simulink model "s_adrc_2"  (R2020b)
settings: Solver=VariableStepAuto  StartTime=0.0  StopTime=10
settings Model: Creator=Amir  LastModifiedBy=Amir
settings DataIOCC: ReturnWorkspaceOutputs=off

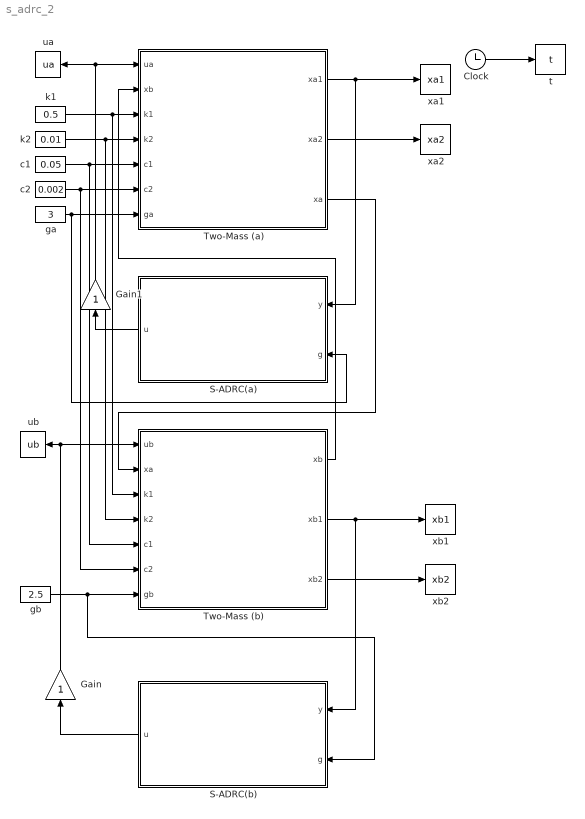
== system s_adrc_2 ==
  Clock : Clock
  Gain : Gain
  Gain1 : Gain
  S-ADRC(a) : Subsystem  mask{alpha1=3, alpha2=3, alpha3=1, epsilon=0.05, xhat0=[1;2;0], p=1, rho=0.5, beta=4, delta=1e+6, deltap=1e+6}
      mask prompts: xhat0 "xhat(0):"; deltap "delta_prime:"
      mask DialogControl ParameterGroupVar Prompt: LESO Parameters
      mask DialogControl ParameterGroupVar_copy Prompt: Controller Parameters
      mask DialogControl ParameterGroupVar_copy_copy Prompt: Thresholds
  S-ADRC(b) : Subsystem  mask{alpha1=3, alpha2=3, alpha3=1, epsilon=0.05, xhat0=[1;2;0], p=1, rho=0.5, beta=4, delta=1e+6, deltap=1e+6}
      mask prompts: xhat0 "xhat(0):"; deltap "delta_prime:"
      mask DialogControl ParameterGroupVar Prompt: LESO Parameters
      mask DialogControl ParameterGroupVar_copy Prompt: Controller Parameters
      mask DialogControl ParameterGroupVar_copy_copy Prompt: Thresholds
  Two-Mass (a) : Subsystem  mask{x0=[1.5;0.5]}
      mask prompts: x0 "x(0):"
  Two-Mass (b) : Subsystem  mask{x0=[1;2]}
      mask prompts: x0 "x(0):"
  c1 : Constant  Value=0.05
  c2 : Constant  Value=0.002
  ga : Constant  Value=3
  gb : Constant  Value=2.5
  k1 : Constant  Value=0.5
  k2 : Constant  Value=0.01
  t : ToWorkspace  VariableName=t  SampleTime=-1
      settings: Save2DSignal=2-D array (concatenate along first dimension)
  ua : ToWorkspace  VariableName=ua  SampleTime=-1
      settings: Save2DSignal=2-D array (concatenate along first dimension)
  ub : ToWorkspace  VariableName=ub  SampleTime=-1
      settings: Save2DSignal=2-D array (concatenate along first dimension)
  xa1 : ToWorkspace  VariableName=xa1  SampleTime=-1
      settings: Save2DSignal=2-D array (concatenate along first dimension)
  xa2 : ToWorkspace  VariableName=xa2  SampleTime=-1
      settings: Save2DSignal=2-D array (concatenate along first dimension)
  xb1 : ToWorkspace  VariableName=xb1  SampleTime=-1
      settings: Save2DSignal=2-D array (concatenate along first dimension)
  xb2 : ToWorkspace  VariableName=xb2  SampleTime=-1
      settings: Save2DSignal=2-D array (concatenate along first dimension)
  wires:
  Two-Mass (a)/2(xa2) -> xa2/1
  Clock/1 -> t/1
  Two-Mass (a)/1(xa1) -> S-ADRC(a)/1(y), xa1/1
  S-ADRC(a)/1(u) -> Gain1/1
  S-ADRC(b)/1(u) -> Gain/1
  Two-Mass (b)/3(xb2) -> xb2/1
  Two-Mass (b)/2(xb1) -> S-ADRC(b)/1(y), xb1/1
  Two-Mass (b)/1(xb) -> Two-Mass (a)/2(xb)
  Two-Mass (a)/3(xa) -> Two-Mass (b)/2(xa)
  k1/1 -> Two-Mass (b)/3(k1), Two-Mass (a)/3(k1)
  k2/1 -> Two-Mass (b)/4(k2), Two-Mass (a)/4(k2)
  c1/1 -> Two-Mass (b)/5(c1), Two-Mass (a)/5(c1)
  c2/1 -> Two-Mass (b)/6(c2), Two-Mass (a)/6(c2)
  ga/1 -> S-ADRC(a)/2(g), Two-Mass (a)/7(ga)
  gb/1 -> S-ADRC(b)/2(g), Two-Mass (b)/7(gb)
  Gain/1 -> Two-Mass (b)/1(ub), ub/1
  Gain1/1 -> Two-Mass (a)/1(ua), ua/1

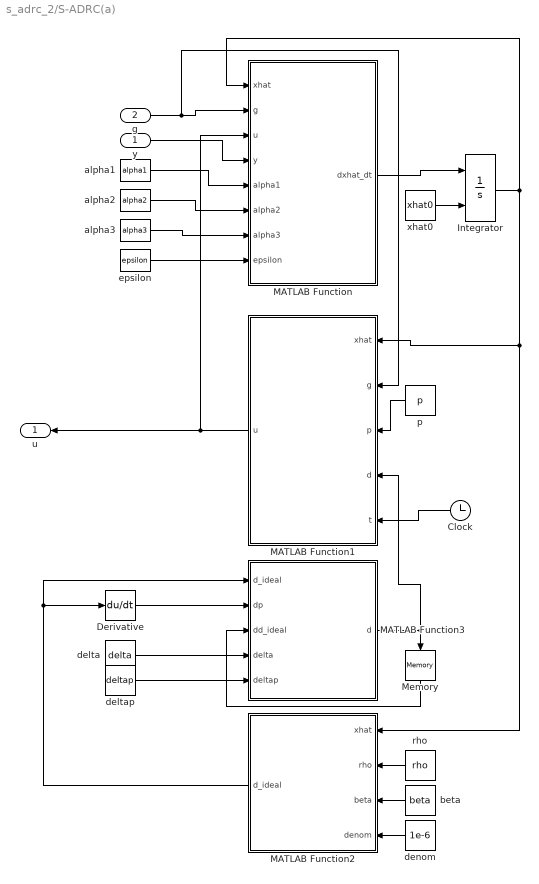
== system s_adrc_2/S-ADRC(a) ==
  y : Inport
  g : Inport  Port=2
  Clock : Clock
  Derivative : Derivative
  Integrator : Integrator  InitialConditionSource=external
  MATLAB Function : MATLAB Function  TreatAsAtomicUnit=on
  MATLAB Function1 : MATLAB Function  TreatAsAtomicUnit=on
  MATLAB Function2 : MATLAB Function  TreatAsAtomicUnit=on
  MATLAB Function3 : MATLAB Function  TreatAsAtomicUnit=on
  Memory : Memory
  alpha1 : Constant  Value=alpha1
  alpha2 : Constant  Value=alpha2
  alpha3 : Constant  Value=alpha3
  beta : Constant  Value=beta
  delta : Constant  Value=delta
  deltap : Constant  Value=deltap
  denom : Constant  Value=1e-6
  epsilon : Constant  Value=epsilon
  p : Constant  Value=p
  rho : Constant  Value=rho
  xhat0 : Constant  Value=xhat0
  u : Outport
  wires:
  Integrator/1 -> MATLAB Function2/1(xhat), MATLAB Function1/1(xhat), MATLAB Function/1(xhat)
  MATLAB Function/1(dxhat_dt) -> Integrator/1
  xhat0/1 -> Integrator/2
  alpha1/1 -> MATLAB Function/5(alpha1)
  alpha2/1 -> MATLAB Function/6(alpha2)
  alpha3/1 -> MATLAB Function/7(alpha3)
  epsilon/1 -> MATLAB Function/8(epsilon)
  y/1 -> MATLAB Function/4(y)
  MATLAB Function1/1(u) -> MATLAB Function/3(u), u/1
  p/1 -> MATLAB Function1/3(p)
  rho/1 -> MATLAB Function2/2(rho)
  beta/1 -> MATLAB Function2/3(beta)
  MATLAB Function3/1(d) -> MATLAB Function1/4(d), Memory/1
  delta/1 -> MATLAB Function3/4(delta)
  deltap/1 -> MATLAB Function3/5(deltap)
  MATLAB Function2/1(d_ideal) -> Derivative/1, MATLAB Function3/1(d_ideal)
  Derivative/1 -> MATLAB Function3/2(dp)
  Memory/1 -> MATLAB Function3/3(dd_ideal)
  denom/1 -> MATLAB Function2/4(denom)
  Clock/1 -> MATLAB Function1/5(t)
  g/1 -> MATLAB Function1/2(g), MATLAB Function/2(g)

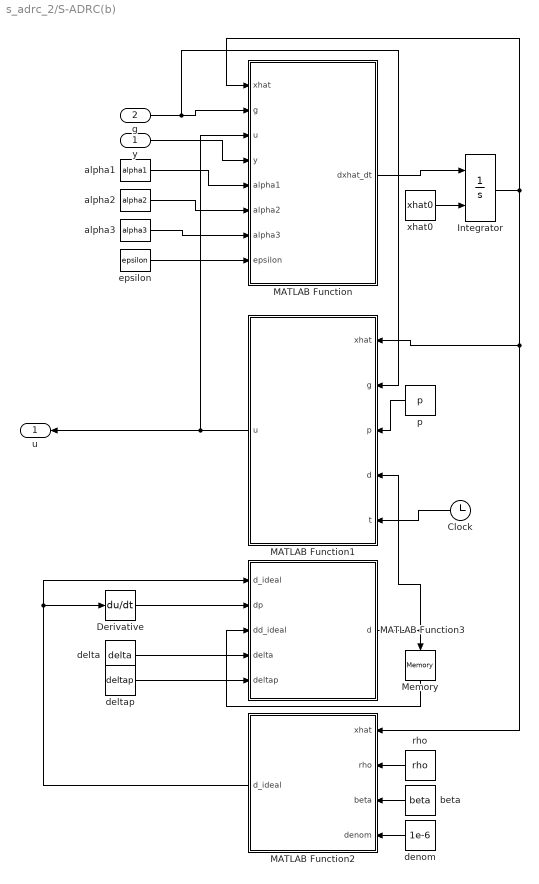
== system s_adrc_2/S-ADRC(b) ==
  y : Inport
  g : Inport  Port=2
  Clock : Clock
  Derivative : Derivative
  Integrator : Integrator  InitialConditionSource=external
  MATLAB Function : MATLAB Function  TreatAsAtomicUnit=on
  MATLAB Function1 : MATLAB Function  TreatAsAtomicUnit=on
  MATLAB Function2 : MATLAB Function  TreatAsAtomicUnit=on
  MATLAB Function3 : MATLAB Function  TreatAsAtomicUnit=on
  Memory : Memory
  alpha1 : Constant  Value=alpha1
  alpha2 : Constant  Value=alpha2
  alpha3 : Constant  Value=alpha3
  beta : Constant  Value=beta
  delta : Constant  Value=delta
  deltap : Constant  Value=deltap
  denom : Constant  Value=1e-6
  epsilon : Constant  Value=epsilon
  p : Constant  Value=p
  rho : Constant  Value=rho
  xhat0 : Constant  Value=xhat0
  u : Outport
  wires:
  Integrator/1 -> MATLAB Function2/1(xhat), MATLAB Function1/1(xhat), MATLAB Function/1(xhat)
  MATLAB Function/1(dxhat_dt) -> Integrator/1
  xhat0/1 -> Integrator/2
  alpha1/1 -> MATLAB Function/5(alpha1)
  alpha2/1 -> MATLAB Function/6(alpha2)
  alpha3/1 -> MATLAB Function/7(alpha3)
  epsilon/1 -> MATLAB Function/8(epsilon)
  y/1 -> MATLAB Function/4(y)
  MATLAB Function1/1(u) -> MATLAB Function/3(u), u/1
  p/1 -> MATLAB Function1/3(p)
  rho/1 -> MATLAB Function2/2(rho)
  beta/1 -> MATLAB Function2/3(beta)
  MATLAB Function3/1(d) -> MATLAB Function1/4(d), Memory/1
  delta/1 -> MATLAB Function3/4(delta)
  deltap/1 -> MATLAB Function3/5(deltap)
  MATLAB Function2/1(d_ideal) -> Derivative/1, MATLAB Function3/1(d_ideal)
  Derivative/1 -> MATLAB Function3/2(dp)
  Memory/1 -> MATLAB Function3/3(dd_ideal)
  denom/1 -> MATLAB Function2/4(denom)
  Clock/1 -> MATLAB Function1/5(t)
  g/1 -> MATLAB Function1/2(g), MATLAB Function/2(g)

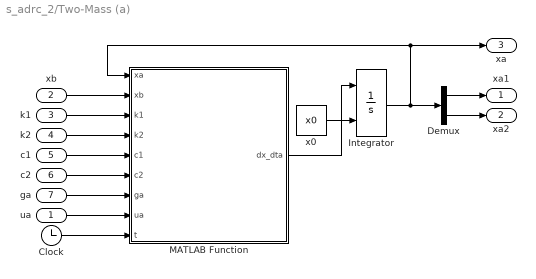
== system s_adrc_2/Two-Mass (a) ==
  ua : Inport
  xb : Inport  Port=2
  k1 : Inport  Port=3
  k2 : Inport  Port=4
  c1 : Inport  Port=5
  c2 : Inport  Port=6
  ga : Inport  Port=7
  Clock : Clock
  Demux : Demux  Outputs=2
  Integrator : Integrator  InitialConditionSource=external
  MATLAB Function : MATLAB Function  TreatAsAtomicUnit=on
  x0 : Constant  Value=x0
  xa1 : Outport
  xa2 : Outport  Port=2
  xa : Outport  Port=3
  wires:
  Integrator/1 -> Demux/1, MATLAB Function/1(xa), xa/1
  MATLAB Function/1(dx_dta) -> Integrator/1
  Demux/1 -> xa1/1
  Demux/2 -> xa2/1
  ua/1 -> MATLAB Function/8(ua)
  Clock/1 -> MATLAB Function/9(t)
  x0/1 -> Integrator/2
  xb/1 -> MATLAB Function/2(xb)
  k2/1 -> MATLAB Function/4(k2)
  k1/1 -> MATLAB Function/3(k1)
  c1/1 -> MATLAB Function/5(c1)
  c2/1 -> MATLAB Function/6(c2)
  ga/1 -> MATLAB Function/7(ga)

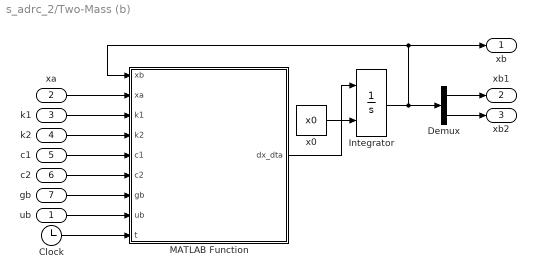
== system s_adrc_2/Two-Mass (b) ==
  ub : Inport
  xa : Inport  Port=2
  k1 : Inport  Port=3
  k2 : Inport  Port=4
  c1 : Inport  Port=5
  c2 : Inport  Port=6
  gb : Inport  Port=7
  Clock : Clock
  Demux : Demux  Outputs=2
  Integrator : Integrator  InitialConditionSource=external
  MATLAB Function : MATLAB Function  TreatAsAtomicUnit=on
  x0 : Constant  Value=x0
  xb : Outport
  xb1 : Outport  Port=2
  xb2 : Outport  Port=3
  wires:
  MATLAB Function/1(dx_dta) -> Integrator/1
  Demux/1 -> xb1/1
  Demux/2 -> xb2/1
  ub/1 -> MATLAB Function/8(ub)
  Clock/1 -> MATLAB Function/9(t)
  x0/1 -> Integrator/2
  k2/1 -> MATLAB Function/4(k2)
  k1/1 -> MATLAB Function/3(k1)
  c1/1 -> MATLAB Function/5(c1)
  c2/1 -> MATLAB Function/6(c2)
  gb/1 -> MATLAB Function/7(gb)
  xa/1 -> MATLAB Function/2(xa)
  Integrator/1 -> MATLAB Function/1(xb), xb/1, Demux/1

== matlab function s_adrc_2/S-ADRC(a)/MATLAB Function2 ==
  data: xhat input; rho input; beta input; d_ideal output; denom input
function d_ideal = d_gen(xhat,rho,beta,denom)

d_ideal=sqrt(((xhat(3)-rho*xhat(1))/(xhat(2)+denom))^2+beta);

== matlab function s_adrc_2/S-ADRC(a)/MATLAB Function3 ==
  data: d_ideal input; dp input; dd_ideal input; d output; delta input; deltap input
function d = d_gen(d_ideal,dp,dd_ideal,delta,deltap)

if d_ideal>delta
    
    d=delta;
    
elseif dd_ideal>deltap
    
    d=dp;
    
else

d = d_ideal;

end

== matlab function s_adrc_2/Two-Mass (b)/MATLAB Function ==
  data: xb input; xa input; k1 input; k2 input; c1 input; c2 input; gb input; ub input; dx_dta output; t input
function dx_dta  = dyn(xb,xa,k1,k2,c1,c2,gb,ub,t)

fb=k1*(xa(1)-xb(1))+k2*(xa(1)-xb(1))^3+c1*(xa(2)-xb(2))+c2*(xa(2)-xb(2))^3;

dx_dta = [xb(2)
         fb+gb*ub];

== matlab function s_adrc_2/S-ADRC(b)/MATLAB Function ==
  data: xhat input; g input; u input; y input; dxhat_dt output; alpha1 input; alpha2 input; alpha3 input; epsilon input
function dxhat_dt = LESO(xhat,g,u,y,alpha1,alpha2,alpha3,epsilon)

dxhat_dt=[xhat(2)+(alpha1/epsilon)*(y-xhat(1))
          xhat(3)+(alpha2/epsilon^2)*(y-xhat(1))+g*u
          (alpha3/epsilon^3)*(y-xhat(1))];

== matlab function s_adrc_2/Two-Mass (a)/MATLAB Function ==
  data: xa input; xb input; k1 input; k2 input; c1 input; c2 input; ga input; ua input; dx_dta output; t input
function dx_dta  = dyn(xa,xb,k1,k2,c1,c2,ga,ua,t)

fb=k1*(xa(1)-xb(1))+k2*(xa(1)-xb(1))^3+c1*(xa(2)-xb(2))+c2*(xa(2)-xb(2))^3;

fa=-fb;

dx_dta = [xa(2)
         fa+ga*ua];

== matlab function s_adrc_2/S-ADRC(b)/MATLAB Function1 ==
  data: xhat input; g input; p input; d input; u output; t input
function u = Controller(xhat,g,p,d,t)

% d=4.2;

u=-1/g*(p*xhat(1)+d*xhat(2)+xhat(3));

if t<0
    
    u=0;
    
end

== matlab function s_adrc_2/S-ADRC(b)/MATLAB Function2 ==
  data: xhat input; rho input; beta input; d_ideal output; denom input
function d_ideal = d_gen(xhat,rho,beta,denom)

d_ideal=sqrt(((xhat(3)-rho*xhat(1))/(xhat(2)+denom))^2+beta);

== matlab function s_adrc_2/S-ADRC(b)/MATLAB Function3 ==
  data: d_ideal input; dp input; dd_ideal input; d output; delta input; deltap input
function d = d_gen(d_ideal,dp,dd_ideal,delta,deltap)

if d_ideal>delta
    
    d=delta;
    
elseif dd_ideal>deltap
    
    d=dp;
    
else

d = d_ideal;

end

== matlab function s_adrc_2/S-ADRC(a)/MATLAB Function ==
  data: xhat input; g input; u input; y input; dxhat_dt output; alpha1 input; alpha2 input; alpha3 input; epsilon input
function dxhat_dt = LESO(xhat,g,u,y,alpha1,alpha2,alpha3,epsilon)

dxhat_dt=[xhat(2)+(alpha1/epsilon)*(y-xhat(1))
          xhat(3)+(alpha2/epsilon^2)*(y-xhat(1))+g*u
          (alpha3/epsilon^3)*(y-xhat(1))];

== matlab function s_adrc_2/S-ADRC(a)/MATLAB Function1 ==
  data: xhat input; g input; p input; d input; u output; t input
function u = Controller(xhat,g,p,d,t)

% d=4.2;

u=-1/g*(p*xhat(1)+d*xhat(2)+xhat(3));

if t<0
    
    u=0;
    
end
